simulink model "Part2B1"  (R2025b)
settings: Solver=VariableStepAuto  StartTime=0.0  StopTime=50  RelTol=1e-3
settings Model: Creator=safiakhalil  LastModifiedBy=safiakhalil

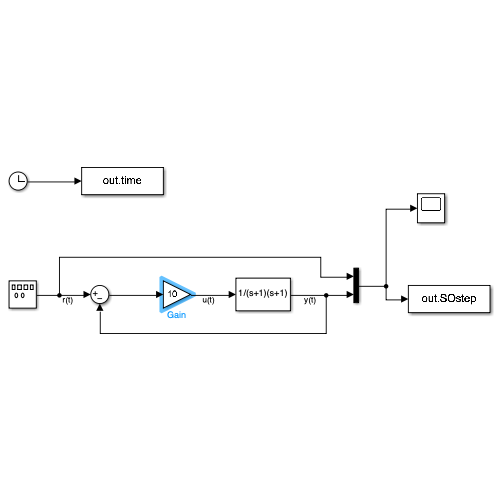
[thumbnail: Simulink's stored preview of the top-level diagram]
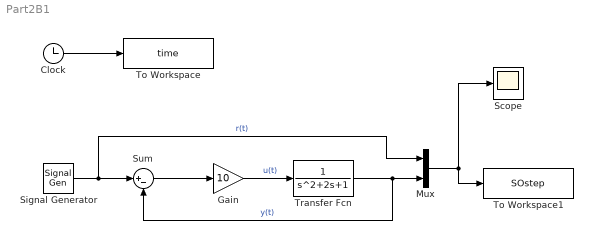
== system Part2B1 ==
  Clock : Clock
  Gain : Gain  Gain=10
  Mux : Mux  Inputs=2
  Scope : Scope
      settings: Title=System Response K=5  ShowGrid=off  ActiveDisplayYMinimum=-1.5462071936560562  ActiveDisplayYMaximum=1.5521113242034237
  Signal Generator : SignalGenerator  WaveForm=square  Frequency=0.05
  Sum : Sum  Inputs=|+-
  To Workspace : ToWorkspace  VariableName=time  SampleTime=-1
  To Workspace1 : ToWorkspace  VariableName=SOstep  SampleTime=-1
  Transfer Fcn : TransferFcn
      mask Display: disp('1/(s+1)(s+1)');
  wires:
  Clock/1 -> To Workspace/1
  Signal Generator/1 -> Mux/1, Sum/1  "r(t)"
  Sum/1 -> Gain/1
  Mux/1 -> To Workspace1/1, Scope/1
  Transfer Fcn/1 -> Sum/2, Mux/2  "y(t)"
  Gain/1 -> Transfer Fcn/1  "u(t)"
